simulink model "OFDM_Tx_Rx_InterpDec"  (R2020a)
settings: Solver=FixedStepDiscrete  StartTime=0.0  StopTime=inf  RelTol=1e-3
InitFcn:
  | % Set parameters
  | fs = 200e3;
  | 
  | % Load all required variables
  | load('read_addr_data');
  | load('read_addr_cp');
  | load('read_addr_pream');
  | load('read_addr_rx');
  | load('pilot');
  | load('LTSfreq');
  | load('STSfreq');
  | load('LTSread');
  | load('STSread');
  | load('bpsk');
  | load('qpsk');
  | load('qam16');
values from neighbouring files (symbols this model uses):
  bpsk = [0 0 1 1 1 1 0 0 1 0 1 0 ... (48 elements, 48x1)]    [bpsk.mat]
  qam16 = [12 5 10 3 14 8 1 10 8 7 2 13 ... (48 elements, 48x1)]    [qam16.mat]
  qpsk = [1 2 1 2 2 2 3 1 1 3 1 0 ... (48 elements, 48x1)]    [qpsk.mat]
  STSfreq = [0 0 0 0 0 0 0 0 1 0 0 0 ... (64 elements, 1x64)]    [STSfreq.mat]
undefined symbols (not defined in the file or in its folder): data3, designMultirateFIR, LTSfreq, LTSread, pilot, read_addr_cp, read_addr_data, read_addr_pream, read_addr_rx, STSread
libraries: hdlsllib x58, simulink x42, dspmlti4 x8, dsphdlxfrm x2, dsphdlmathfun x2, dsphdlsigops x1
(part 4 of 5)

== system OFDM_Tx_Rx_InterpDec/OFDMRx/Synchronisation/FineTimingSynch/MatchedFilter/Adder22 ==
  In1 : Inport
  In2 : Inport  Port=2
  Add : Sum  AccumDataTypeStr=fixdt(1,24,14)
  Delay3 : Delay  DelayLength=1
  Out1 : Outport  VectorParamsAs1DForOutWhenUnconnected=off
  wires:
  In2/1 -> Delay3/1
  In1/1 -> Add/1
  Add/1 -> Out1/1
  Delay3/1 -> Add/2

== system OFDM_Tx_Rx_InterpDec/OFDMRx/Synchronisation/FineTimingSynch/MatchedFilter/Adder23 ==
  In1 : Inport
  In2 : Inport  Port=2
  Add : Sum  AccumDataTypeStr=fixdt(1,24,14)
  Delay3 : Delay  DelayLength=1
  Out1 : Outport  VectorParamsAs1DForOutWhenUnconnected=off
  wires:
  In2/1 -> Delay3/1
  In1/1 -> Add/1
  Add/1 -> Out1/1
  Delay3/1 -> Add/2

== system OFDM_Tx_Rx_InterpDec/OFDMRx/Synchronisation/FineTimingSynch/MatchedFilter/Adder24 ==
  In1 : Inport
  In2 : Inport  Port=2
  Add : Sum  AccumDataTypeStr=fixdt(1,24,14)
  Delay3 : Delay  DelayLength=1
  Out1 : Outport  VectorParamsAs1DForOutWhenUnconnected=off
  wires:
  In2/1 -> Delay3/1
  In1/1 -> Add/1
  Add/1 -> Out1/1
  Delay3/1 -> Add/2

== system OFDM_Tx_Rx_InterpDec/OFDMRx/Synchronisation/FineTimingSynch/MatchedFilter/Adder25 ==
  In1 : Inport
  In2 : Inport  Port=2
  Add : Sum  AccumDataTypeStr=fixdt(1,24,14)
  Delay3 : Delay  DelayLength=1
  Out1 : Outport  VectorParamsAs1DForOutWhenUnconnected=off
  wires:
  In2/1 -> Delay3/1
  In1/1 -> Add/1
  Add/1 -> Out1/1
  Delay3/1 -> Add/2

== system OFDM_Tx_Rx_InterpDec/OFDMRx/Synchronisation/FineTimingSynch/MatchedFilter/Adder26 ==
  In1 : Inport
  In2 : Inport  Port=2
  Add : Sum  AccumDataTypeStr=fixdt(1,24,14)
  Delay3 : Delay  DelayLength=1
  Out1 : Outport  VectorParamsAs1DForOutWhenUnconnected=off
  wires:
  In2/1 -> Delay3/1
  In1/1 -> Add/1
  Add/1 -> Out1/1
  Delay3/1 -> Add/2

== system OFDM_Tx_Rx_InterpDec/OFDMRx/Synchronisation/FineTimingSynch/MatchedFilter/Adder27 ==
  In1 : Inport
  In2 : Inport  Port=2
  Add : Sum  AccumDataTypeStr=fixdt(1,24,14)
  Delay3 : Delay  DelayLength=1
  Out1 : Outport  VectorParamsAs1DForOutWhenUnconnected=off
  wires:
  In2/1 -> Delay3/1
  In1/1 -> Add/1
  Add/1 -> Out1/1
  Delay3/1 -> Add/2

== system OFDM_Tx_Rx_InterpDec/OFDMRx/Synchronisation/FineTimingSynch/MatchedFilter/Adder28 ==
  In1 : Inport
  In2 : Inport  Port=2
  Add : Sum
  Delay3 : Delay  DelayLength=1
  Out1 : Outport  VectorParamsAs1DForOutWhenUnconnected=off
  wires:
  In2/1 -> Delay3/1
  In1/1 -> Add/1
  Add/1 -> Out1/1
  Delay3/1 -> Add/2

== system OFDM_Tx_Rx_InterpDec/OFDMRx/Synchronisation/FineTimingSynch/MatchedFilter/Adder29 ==
  In1 : Inport
  In2 : Inport  Port=2
  Add : Sum  AccumDataTypeStr=fixdt(1,24,14)
  Delay3 : Delay  DelayLength=1
  Out1 : Outport  VectorParamsAs1DForOutWhenUnconnected=off
  wires:
  In2/1 -> Delay3/1
  In1/1 -> Add/1
  Add/1 -> Out1/1
  Delay3/1 -> Add/2

== system OFDM_Tx_Rx_InterpDec/OFDMRx/Synchronisation/FineTimingSynch/MatchedFilter/Adder3 ==
  In1 : Inport
  In2 : Inport  Port=2
  Add : Sum  AccumDataTypeStr=fixdt(1,24,14)
  Delay3 : Delay  DelayLength=1
  Out1 : Outport  VectorParamsAs1DForOutWhenUnconnected=off
  wires:
  Delay3/1 -> Add/2
  Add/1 -> Out1/1
  In1/1 -> Add/1
  In2/1 -> Delay3/1

== system OFDM_Tx_Rx_InterpDec/OFDMRx/Synchronisation/FineTimingSynch/MatchedFilter/Adder30 ==
  In1 : Inport
  In2 : Inport  Port=2
  Add : Sum  AccumDataTypeStr=fixdt(1,24,14)
  Delay3 : Delay  DelayLength=1
  Out1 : Outport  VectorParamsAs1DForOutWhenUnconnected=off
  wires:
  In2/1 -> Delay3/1
  In1/1 -> Add/1
  Add/1 -> Out1/1
  Delay3/1 -> Add/2

== system OFDM_Tx_Rx_InterpDec/OFDMRx/Synchronisation/FineTimingSynch/MatchedFilter/Adder31 ==
  In1 : Inport
  In2 : Inport  Port=2
  Add : Sum  AccumDataTypeStr=fixdt(1,24,14)
  Delay3 : Delay  DelayLength=1
  Out1 : Outport  VectorParamsAs1DForOutWhenUnconnected=off
  wires:
  In2/1 -> Delay3/1
  In1/1 -> Add/1
  Add/1 -> Out1/1
  Delay3/1 -> Add/2

== system OFDM_Tx_Rx_InterpDec/OFDMRx/Synchronisation/FineTimingSynch/MatchedFilter/Adder32 ==
  In1 : Inport
  In2 : Inport  Port=2
  Add : Sum  AccumDataTypeStr=fixdt(1,24,14)
  Delay3 : Delay  DelayLength=1
  Out1 : Outport  VectorParamsAs1DForOutWhenUnconnected=off
  wires:
  In2/1 -> Delay3/1
  In1/1 -> Add/1
  Add/1 -> Out1/1
  Delay3/1 -> Add/2

== system OFDM_Tx_Rx_InterpDec/OFDMRx/Synchronisation/FineTimingSynch/MatchedFilter/Adder33 ==
  In1 : Inport
  In2 : Inport  Port=2
  Add : Sum  AccumDataTypeStr=fixdt(1,24,14)
  Delay3 : Delay  DelayLength=1
  Out1 : Outport  VectorParamsAs1DForOutWhenUnconnected=off
  wires:
  In2/1 -> Delay3/1
  In1/1 -> Add/1
  Add/1 -> Out1/1
  Delay3/1 -> Add/2

== system OFDM_Tx_Rx_InterpDec/OFDMRx/Synchronisation/FineTimingSynch/MatchedFilter/Adder34 ==
  In1 : Inport
  In2 : Inport  Port=2
  Add : Sum  AccumDataTypeStr=fixdt(1,24,14)
  Delay3 : Delay  DelayLength=1
  Out1 : Outport  VectorParamsAs1DForOutWhenUnconnected=off
  wires:
  In2/1 -> Delay3/1
  In1/1 -> Add/1
  Add/1 -> Out1/1
  Delay3/1 -> Add/2

== system OFDM_Tx_Rx_InterpDec/OFDMRx/Synchronisation/FineTimingSynch/MatchedFilter/Adder35 ==
  In1 : Inport
  In2 : Inport  Port=2
  Add : Sum  AccumDataTypeStr=fixdt(1,24,14)
  Delay3 : Delay  DelayLength=1
  Out1 : Outport  VectorParamsAs1DForOutWhenUnconnected=off
  wires:
  In2/1 -> Delay3/1
  In1/1 -> Add/1
  Add/1 -> Out1/1
  Delay3/1 -> Add/2

== system OFDM_Tx_Rx_InterpDec/OFDMRx/Synchronisation/FineTimingSynch/MatchedFilter/Adder36 ==
  In1 : Inport
  In2 : Inport  Port=2
  Add : Sum  AccumDataTypeStr=fixdt(1,24,14)
  Delay3 : Delay  DelayLength=1
  Out1 : Outport  VectorParamsAs1DForOutWhenUnconnected=off
  wires:
  In2/1 -> Delay3/1
  In1/1 -> Add/1
  Add/1 -> Out1/1
  Delay3/1 -> Add/2

== system OFDM_Tx_Rx_InterpDec/OFDMRx/Synchronisation/FineTimingSynch/MatchedFilter/Adder37 ==
  In1 : Inport
  In2 : Inport  Port=2
  Add : Sum  AccumDataTypeStr=fixdt(1,24,14)
  Delay3 : Delay  DelayLength=1
  Out1 : Outport  VectorParamsAs1DForOutWhenUnconnected=off
  wires:
  In2/1 -> Delay3/1
  In1/1 -> Add/1
  Add/1 -> Out1/1
  Delay3/1 -> Add/2

== system OFDM_Tx_Rx_InterpDec/OFDMRx/Synchronisation/FineTimingSynch/MatchedFilter/Adder38 ==
  In1 : Inport
  In2 : Inport  Port=2
  Add : Sum  AccumDataTypeStr=fixdt(1,24,14)
  Delay3 : Delay  DelayLength=1
  Out1 : Outport  VectorParamsAs1DForOutWhenUnconnected=off
  wires:
  In2/1 -> Delay3/1
  In1/1 -> Add/1
  Add/1 -> Out1/1
  Delay3/1 -> Add/2

== system OFDM_Tx_Rx_InterpDec/OFDMRx/Synchronisation/FineTimingSynch/MatchedFilter/Adder39 ==
  In1 : Inport
  In2 : Inport  Port=2
  Add : Sum  AccumDataTypeStr=fixdt(1,24,14)
  Delay3 : Delay  DelayLength=1
  Out1 : Outport  VectorParamsAs1DForOutWhenUnconnected=off
  wires:
  In2/1 -> Delay3/1
  In1/1 -> Add/1
  Add/1 -> Out1/1
  Delay3/1 -> Add/2

== system OFDM_Tx_Rx_InterpDec/OFDMRx/Synchronisation/FineTimingSynch/MatchedFilter/Adder4 ==
  In1 : Inport
  In2 : Inport  Port=2
  Add : Sum  AccumDataTypeStr=fixdt(1,24,14)
  Delay3 : Delay  DelayLength=1
  Out1 : Outport  VectorParamsAs1DForOutWhenUnconnected=off
  wires:
  In2/1 -> Delay3/1
  In1/1 -> Add/1
  Add/1 -> Out1/1
  Delay3/1 -> Add/2

== system OFDM_Tx_Rx_InterpDec/OFDMRx/Synchronisation/FineTimingSynch/MatchedFilter/Adder40 ==
  In1 : Inport
  In2 : Inport  Port=2
  Add : Sum  AccumDataTypeStr=fixdt(1,24,14)
  Delay3 : Delay  DelayLength=1
  Out1 : Outport  VectorParamsAs1DForOutWhenUnconnected=off
  wires:
  In2/1 -> Delay3/1
  In1/1 -> Add/1
  Add/1 -> Out1/1
  Delay3/1 -> Add/2

== system OFDM_Tx_Rx_InterpDec/OFDMRx/Synchronisation/FineTimingSynch/MatchedFilter/Adder41 ==
  In1 : Inport
  In2 : Inport  Port=2
  Add : Sum  AccumDataTypeStr=fixdt(1,24,14)
  Delay3 : Delay  DelayLength=1
  Out1 : Outport  VectorParamsAs1DForOutWhenUnconnected=off
  wires:
  In2/1 -> Delay3/1
  In1/1 -> Add/1
  Add/1 -> Out1/1
  Delay3/1 -> Add/2

== system OFDM_Tx_Rx_InterpDec/OFDMRx/Synchronisation/FineTimingSynch/MatchedFilter/Adder42 ==
  In1 : Inport
  In2 : Inport  Port=2
  Add : Sum  AccumDataTypeStr=fixdt(1,24,14)
  Delay3 : Delay  DelayLength=1
  Out1 : Outport  VectorParamsAs1DForOutWhenUnconnected=off
  wires:
  In2/1 -> Delay3/1
  In1/1 -> Add/1
  Add/1 -> Out1/1
  Delay3/1 -> Add/2

== system OFDM_Tx_Rx_InterpDec/OFDMRx/Synchronisation/FineTimingSynch/MatchedFilter/Adder43 ==
  In1 : Inport
  In2 : Inport  Port=2
  Add : Sum  AccumDataTypeStr=fixdt(1,24,14)
  Delay3 : Delay  DelayLength=1
  Out1 : Outport  VectorParamsAs1DForOutWhenUnconnected=off
  wires:
  In2/1 -> Delay3/1
  In1/1 -> Add/1
  Add/1 -> Out1/1
  Delay3/1 -> Add/2

== system OFDM_Tx_Rx_InterpDec/OFDMRx/Synchronisation/FineTimingSynch/MatchedFilter/Adder44 ==
  In1 : Inport
  In2 : Inport  Port=2
  Add : Sum  AccumDataTypeStr=fixdt(1,24,14)
  Delay3 : Delay  DelayLength=1
  Out1 : Outport  VectorParamsAs1DForOutWhenUnconnected=off
  wires:
  In2/1 -> Delay3/1
  In1/1 -> Add/1
  Add/1 -> Out1/1
  Delay3/1 -> Add/2

== system OFDM_Tx_Rx_InterpDec/OFDMRx/Synchronisation/FineTimingSynch/MatchedFilter/Adder45 ==
  In1 : Inport
  In2 : Inport  Port=2
  Add : Sum  AccumDataTypeStr=fixdt(1,24,14)
  Delay3 : Delay  DelayLength=1
  Out1 : Outport  VectorParamsAs1DForOutWhenUnconnected=off
  wires:
  In2/1 -> Delay3/1
  In1/1 -> Add/1
  Add/1 -> Out1/1
  Delay3/1 -> Add/2

== system OFDM_Tx_Rx_InterpDec/OFDMRx/Synchronisation/FineTimingSynch/MatchedFilter/Adder46 ==
  In1 : Inport
  In2 : Inport  Port=2
  Add : Sum  AccumDataTypeStr=fixdt(1,24,14)
  Delay3 : Delay  DelayLength=1
  Out1 : Outport  VectorParamsAs1DForOutWhenUnconnected=off
  wires:
  In2/1 -> Delay3/1
  In1/1 -> Add/1
  Add/1 -> Out1/1
  Delay3/1 -> Add/2

== system OFDM_Tx_Rx_InterpDec/OFDMRx/Synchronisation/FineTimingSynch/MatchedFilter/Adder47 ==
  In1 : Inport
  In2 : Inport  Port=2
  Add : Sum  AccumDataTypeStr=fixdt(1,24,14)
  Delay3 : Delay  DelayLength=1
  Out1 : Outport  VectorParamsAs1DForOutWhenUnconnected=off
  wires:
  In2/1 -> Delay3/1
  In1/1 -> Add/1
  Add/1 -> Out1/1
  Delay3/1 -> Add/2

== system OFDM_Tx_Rx_InterpDec/OFDMRx/Synchronisation/FineTimingSynch/MatchedFilter/Adder48 ==
  In1 : Inport
  In2 : Inport  Port=2
  Add : Sum  AccumDataTypeStr=fixdt(1,24,14)
  Delay3 : Delay  DelayLength=1
  Out1 : Outport  VectorParamsAs1DForOutWhenUnconnected=off
  wires:
  In2/1 -> Delay3/1
  In1/1 -> Add/1
  Add/1 -> Out1/1
  Delay3/1 -> Add/2

== system OFDM_Tx_Rx_InterpDec/OFDMRx/Synchronisation/FineTimingSynch/MatchedFilter/Adder49 ==
  In1 : Inport
  In2 : Inport  Port=2
  Add : Sum  AccumDataTypeStr=fixdt(1,24,14)
  Delay3 : Delay  DelayLength=1
  Out1 : Outport  VectorParamsAs1DForOutWhenUnconnected=off
  wires:
  In2/1 -> Delay3/1
  In1/1 -> Add/1
  Add/1 -> Out1/1
  Delay3/1 -> Add/2

== system OFDM_Tx_Rx_InterpDec/OFDMRx/Synchronisation/FineTimingSynch/MatchedFilter/Adder5 ==
  In1 : Inport
  In2 : Inport  Port=2
  Add : Sum  AccumDataTypeStr=fixdt(1,24,14)
  Delay3 : Delay  DelayLength=1
  Out1 : Outport  VectorParamsAs1DForOutWhenUnconnected=off
  wires:
  Delay3/1 -> Add/2
  Add/1 -> Out1/1
  In1/1 -> Add/1
  In2/1 -> Delay3/1

== system OFDM_Tx_Rx_InterpDec/OFDMRx/Synchronisation/FineTimingSynch/MatchedFilter/Adder50 ==
  In1 : Inport
  In2 : Inport  Port=2
  Add : Sum  AccumDataTypeStr=fixdt(1,24,14)
  Delay3 : Delay  DelayLength=1
  Out1 : Outport  VectorParamsAs1DForOutWhenUnconnected=off
  wires:
  In2/1 -> Delay3/1
  In1/1 -> Add/1
  Add/1 -> Out1/1
  Delay3/1 -> Add/2

== system OFDM_Tx_Rx_InterpDec/OFDMRx/Synchronisation/FineTimingSynch/MatchedFilter/Adder51 ==
  In1 : Inport
  In2 : Inport  Port=2
  Add : Sum  AccumDataTypeStr=fixdt(1,24,14)
  Delay3 : Delay  DelayLength=1
  Out1 : Outport  VectorParamsAs1DForOutWhenUnconnected=off
  wires:
  In2/1 -> Delay3/1
  In1/1 -> Add/1
  Add/1 -> Out1/1
  Delay3/1 -> Add/2

== system OFDM_Tx_Rx_InterpDec/OFDMRx/Synchronisation/FineTimingSynch/MatchedFilter/Adder52 ==
  In1 : Inport
  In2 : Inport  Port=2
  Add : Sum  AccumDataTypeStr=fixdt(1,24,14)
  Delay3 : Delay  DelayLength=1
  Out1 : Outport  VectorParamsAs1DForOutWhenUnconnected=off
  wires:
  In2/1 -> Delay3/1
  In1/1 -> Add/1
  Add/1 -> Out1/1
  Delay3/1 -> Add/2

== system OFDM_Tx_Rx_InterpDec/OFDMRx/Synchronisation/FineTimingSynch/MatchedFilter/Adder53 ==
  In1 : Inport
  In2 : Inport  Port=2
  Add : Sum  AccumDataTypeStr=fixdt(1,24,14)
  Delay3 : Delay  DelayLength=1
  Out1 : Outport  VectorParamsAs1DForOutWhenUnconnected=off
  wires:
  In2/1 -> Delay3/1
  In1/1 -> Add/1
  Add/1 -> Out1/1
  Delay3/1 -> Add/2

== system OFDM_Tx_Rx_InterpDec/OFDMRx/Synchronisation/FineTimingSynch/MatchedFilter/Adder54 ==
  In1 : Inport
  In2 : Inport  Port=2
  Add : Sum  AccumDataTypeStr=fixdt(1,24,14)
  Delay3 : Delay  DelayLength=1
  Out1 : Outport  VectorParamsAs1DForOutWhenUnconnected=off
  wires:
  In2/1 -> Delay3/1
  In1/1 -> Add/1
  Add/1 -> Out1/1
  Delay3/1 -> Add/2

== system OFDM_Tx_Rx_InterpDec/OFDMRx/Synchronisation/FineTimingSynch/MatchedFilter/Adder55 ==
  In1 : Inport
  In2 : Inport  Port=2
  Add : Sum  AccumDataTypeStr=fixdt(1,24,14)
  Delay3 : Delay  DelayLength=1
  Out1 : Outport  VectorParamsAs1DForOutWhenUnconnected=off
  wires:
  In2/1 -> Delay3/1
  In1/1 -> Add/1
  Add/1 -> Out1/1
  Delay3/1 -> Add/2

== system OFDM_Tx_Rx_InterpDec/OFDMRx/Synchronisation/FineTimingSynch/MatchedFilter/Adder56 ==
  In1 : Inport
  In2 : Inport  Port=2
  Add : Sum  AccumDataTypeStr=fixdt(1,24,14)
  Delay3 : Delay  DelayLength=1
  Out1 : Outport  VectorParamsAs1DForOutWhenUnconnected=off
  wires:
  In2/1 -> Delay3/1
  In1/1 -> Add/1
  Add/1 -> Out1/1
  Delay3/1 -> Add/2

== system OFDM_Tx_Rx_InterpDec/OFDMRx/Synchronisation/FineTimingSynch/MatchedFilter/Adder57 ==
  In1 : Inport
  In2 : Inport  Port=2
  Add : Sum  AccumDataTypeStr=fixdt(1,24,14)
  Delay3 : Delay  DelayLength=1
  Out1 : Outport  VectorParamsAs1DForOutWhenUnconnected=off
  wires:
  In2/1 -> Delay3/1
  In1/1 -> Add/1
  Add/1 -> Out1/1
  Delay3/1 -> Add/2

== system OFDM_Tx_Rx_InterpDec/OFDMRx/Synchronisation/FineTimingSynch/MatchedFilter/Adder58 ==
  In1 : Inport
  In2 : Inport  Port=2
  Add : Sum  AccumDataTypeStr=fixdt(1,24,14)
  Delay3 : Delay  DelayLength=1
  Out1 : Outport  VectorParamsAs1DForOutWhenUnconnected=off
  wires:
  In2/1 -> Delay3/1
  In1/1 -> Add/1
  Add/1 -> Out1/1
  Delay3/1 -> Add/2

== system OFDM_Tx_Rx_InterpDec/OFDMRx/Synchronisation/FineTimingSynch/MatchedFilter/Adder59 ==
  In1 : Inport
  In2 : Inport  Port=2
  Add : Sum  AccumDataTypeStr=fixdt(1,24,14)
  Delay3 : Delay  DelayLength=1
  Out1 : Outport  VectorParamsAs1DForOutWhenUnconnected=off
  wires:
  In2/1 -> Delay3/1
  In1/1 -> Add/1
  Add/1 -> Out1/1
  Delay3/1 -> Add/2

== system OFDM_Tx_Rx_InterpDec/OFDMRx/Synchronisation/FineTimingSynch/MatchedFilter/Adder6 ==
  In1 : Inport
  In2 : Inport  Port=2
  Add : Sum  AccumDataTypeStr=fixdt(1,24,14)
  Delay3 : Delay  DelayLength=1
  Out1 : Outport  VectorParamsAs1DForOutWhenUnconnected=off
  wires:
  In2/1 -> Delay3/1
  In1/1 -> Add/1
  Add/1 -> Out1/1
  Delay3/1 -> Add/2

== system OFDM_Tx_Rx_InterpDec/OFDMRx/Synchronisation/FineTimingSynch/MatchedFilter/Adder60 ==
  In1 : Inport
  In2 : Inport  Port=2
  Add : Sum  AccumDataTypeStr=fixdt(1,24,14)
  Delay3 : Delay  DelayLength=1
  Out1 : Outport  VectorParamsAs1DForOutWhenUnconnected=off
  wires:
  In2/1 -> Delay3/1
  In1/1 -> Add/1
  Add/1 -> Out1/1
  Delay3/1 -> Add/2

== system OFDM_Tx_Rx_InterpDec/OFDMRx/Synchronisation/FineTimingSynch/MatchedFilter/Adder61 ==
  In1 : Inport
  In2 : Inport  Port=2
  Add : Sum  AccumDataTypeStr=fixdt(1,24,14)
  Delay3 : Delay  DelayLength=1
  Out1 : Outport  VectorParamsAs1DForOutWhenUnconnected=off
  wires:
  In2/1 -> Delay3/1
  In1/1 -> Add/1
  Add/1 -> Out1/1
  Delay3/1 -> Add/2

== system OFDM_Tx_Rx_InterpDec/OFDMRx/Synchronisation/FineTimingSynch/MatchedFilter/Adder62 ==
  In1 : Inport
  In2 : Inport  Port=2
  Add : Sum  AccumDataTypeStr=fixdt(1,24,14)
  Delay3 : Delay  DelayLength=1
  Out1 : Outport  VectorParamsAs1DForOutWhenUnconnected=off
  wires:
  In2/1 -> Delay3/1
  In1/1 -> Add/1
  Add/1 -> Out1/1
  Delay3/1 -> Add/2

== system OFDM_Tx_Rx_InterpDec/OFDMRx/Synchronisation/FineTimingSynch/MatchedFilter/Adder7 ==
  In1 : Inport
  In2 : Inport  Port=2
  Add : Sum  AccumDataTypeStr=fixdt(1,24,14)
  Delay3 : Delay  DelayLength=1
  Out1 : Outport  VectorParamsAs1DForOutWhenUnconnected=off
  wires:
  Delay3/1 -> Add/2
  Add/1 -> Out1/1
  In1/1 -> Add/1
  In2/1 -> Delay3/1

== system OFDM_Tx_Rx_InterpDec/OFDMRx/Synchronisation/FineTimingSynch/MatchedFilter/Adder8 ==
  In1 : Inport
  In2 : Inport  Port=2
  Add : Sum  AccumDataTypeStr=fixdt(1,24,14)
  Delay3 : Delay  DelayLength=1
  Out1 : Outport  VectorParamsAs1DForOutWhenUnconnected=off
  wires:
  In2/1 -> Delay3/1
  In1/1 -> Add/1
  Add/1 -> Out1/1
  Delay3/1 -> Add/2

== system OFDM_Tx_Rx_InterpDec/OFDMRx/Synchronisation/FineTimingSynch/MatchedFilter/Adder9 ==
  In1 : Inport
  In2 : Inport  Port=2
  Add : Sum  AccumDataTypeStr=fixdt(1,24,14)
  Delay3 : Delay  DelayLength=1
  Out1 : Outport  VectorParamsAs1DForOutWhenUnconnected=off
  wires:
  Delay3/1 -> Add/2
  Add/1 -> Out1/1
  In1/1 -> Add/1
  In2/1 -> Delay3/1

== system OFDM_Tx_Rx_InterpDec/OFDMRx/Synchronisation/FineTimingSynch/MatchedFilter/Subsystem ==
  MatchedIn : Inport
  Add : Sum  OutDataTypeStr=fixdt(1,18,14)
  Add1 : Sum  Inputs=+-  OutDataTypeStr=fixdt(1,18,14)
  Complex to Real-Imag : ComplexToRealImag
  Real-Imag to Complex : RealImagToComplex
  Unary Minus : UnaryMinus
  Out1 : Outport
  wires:
  Real-Imag to Complex/1 -> Out1/1
  MatchedIn/1 -> Complex to Real-Imag/1
  Add1/1 -> Real-Imag to Complex/1
  Complex to Real-Imag/2 -> Add/2, Add1/1
  Complex to Real-Imag/1 -> Add/1, Add1/2
  Add/1 -> Unary Minus/1
  Unary Minus/1 -> Real-Imag to Complex/2

== system OFDM_Tx_Rx_InterpDec/OFDMRx/Synchronisation/FineTimingSynch/MatchedFilter/Subsystem1 ==
  MatchedIn : Inport
  Add : Sum  OutDataTypeStr=fixdt(1,18,14)
  Add1 : Sum  Inputs=+-  OutDataTypeStr=fixdt(1,18,14)
  Complex to Real-Imag : ComplexToRealImag
  Real-Imag to Complex : RealImagToComplex
  Out1 : Outport
  wires:
  Complex to Real-Imag/2 -> Add1/1, Add/2
  Add/1 -> Real-Imag to Complex/1
  Add1/1 -> Real-Imag to Complex/2
  Complex to Real-Imag/1 -> Add1/2, Add/1
  MatchedIn/1 -> Complex to Real-Imag/1
  Real-Imag to Complex/1 -> Out1/1

== system OFDM_Tx_Rx_InterpDec/OFDMRx/Synchronisation/FineTimingSynch/MatchedFilter/Subsystem10 ==
  MatchedIn : Inport
  Add : Sum  OutDataTypeStr=fixdt(1,18,14)
  Add1 : Sum  Inputs=+-  OutDataTypeStr=fixdt(1,18,14)
  Complex to Real-Imag : ComplexToRealImag
  Real-Imag to Complex : RealImagToComplex
  Unary Minus : UnaryMinus
  Out1 : Outport
  wires:
  Unary Minus/1 -> Real-Imag to Complex/2
  Add/1 -> Unary Minus/1
  Complex to Real-Imag/1 -> Add1/2, Add/1
  Complex to Real-Imag/2 -> Add1/1, Add/2
  Add1/1 -> Real-Imag to Complex/1
  MatchedIn/1 -> Complex to Real-Imag/1
  Real-Imag to Complex/1 -> Out1/1

== system OFDM_Tx_Rx_InterpDec/OFDMRx/Synchronisation/FineTimingSynch/MatchedFilter/Subsystem11 ==
  MatchedIn : Inport
  Add : Sum  OutDataTypeStr=fixdt(1,18,14)
  Add1 : Sum  Inputs=+-  OutDataTypeStr=fixdt(1,18,14)
  Complex to Real-Imag : ComplexToRealImag
  Real-Imag to Complex : RealImagToComplex
  Out1 : Outport
  wires:
  Real-Imag to Complex/1 -> Out1/1
  MatchedIn/1 -> Complex to Real-Imag/1
  Complex to Real-Imag/1 -> Add/1, Add1/2
  Add1/1 -> Real-Imag to Complex/2
  Add/1 -> Real-Imag to Complex/1
  Complex to Real-Imag/2 -> Add/2, Add1/1

== system OFDM_Tx_Rx_InterpDec/OFDMRx/Synchronisation/FineTimingSynch/MatchedFilter/Subsystem12 ==
  MatchedIn : Inport
  Add : Sum  OutDataTypeStr=fixdt(1,18,14)
  Add1 : Sum  Inputs=+-  OutDataTypeStr=fixdt(1,18,14)
  Complex to Real-Imag : ComplexToRealImag
  Real-Imag to Complex : RealImagToComplex
  Out1 : Outport
  wires:
  Real-Imag to Complex/1 -> Out1/1
  MatchedIn/1 -> Complex to Real-Imag/1
  Complex to Real-Imag/1 -> Add/1, Add1/2
  Add1/1 -> Real-Imag to Complex/2
  Add/1 -> Real-Imag to Complex/1
  Complex to Real-Imag/2 -> Add/2, Add1/1

== system OFDM_Tx_Rx_InterpDec/OFDMRx/Synchronisation/FineTimingSynch/MatchedFilter/Subsystem13 ==
  MatchedIn : Inport
  Add : Sum  OutDataTypeStr=fixdt(1,18,14)
  Add1 : Sum  Inputs=+-  OutDataTypeStr=fixdt(1,18,14)
  Complex to Real-Imag : ComplexToRealImag
  Real-Imag to Complex : RealImagToComplex
  Unary Minus : UnaryMinus
  Out1 : Outport
  wires:
  Complex to Real-Imag/2 -> Add1/2, Add/2
  Add/1 -> Unary Minus/1
  Add1/1 -> Real-Imag to Complex/2
  Complex to Real-Imag/1 -> Add1/1, Add/1
  MatchedIn/1 -> Complex to Real-Imag/1
  Real-Imag to Complex/1 -> Out1/1
  Unary Minus/1 -> Real-Imag to Complex/1

== system OFDM_Tx_Rx_InterpDec/OFDMRx/Synchronisation/FineTimingSynch/MatchedFilter/Subsystem14 ==
  MatchedIn : Inport
  Add : Sum  OutDataTypeStr=fixdt(1,18,14)
  Add1 : Sum  Inputs=+-  OutDataTypeStr=fixdt(1,18,14)
  Complex to Real-Imag : ComplexToRealImag
  Real-Imag to Complex : RealImagToComplex
  Out1 : Outport
  wires:
  Real-Imag to Complex/1 -> Out1/1
  MatchedIn/1 -> Complex to Real-Imag/1
  Complex to Real-Imag/1 -> Add/1, Add1/2
  Add1/1 -> Real-Imag to Complex/2
  Add/1 -> Real-Imag to Complex/1
  Complex to Real-Imag/2 -> Add/2, Add1/1

== system OFDM_Tx_Rx_InterpDec/OFDMRx/Synchronisation/FineTimingSynch/MatchedFilter/Subsystem15 ==
  MatchedIn : Inport
  Add : Sum  OutDataTypeStr=fixdt(1,18,14)
  Add1 : Sum  Inputs=+-  OutDataTypeStr=fixdt(1,18,14)
  Complex to Real-Imag : ComplexToRealImag
  Real-Imag to Complex : RealImagToComplex
  Out1 : Outport
  wires:
  Real-Imag to Complex/1 -> Out1/1
  MatchedIn/1 -> Complex to Real-Imag/1
  Complex to Real-Imag/1 -> Add/1, Add1/2
  Add1/1 -> Real-Imag to Complex/2
  Add/1 -> Real-Imag to Complex/1
  Complex to Real-Imag/2 -> Add/2, Add1/1

== system OFDM_Tx_Rx_InterpDec/OFDMRx/Synchronisation/FineTimingSynch/MatchedFilter/Subsystem16 ==
  MatchedIn : Inport
  Add : Sum  OutDataTypeStr=fixdt(1,18,14)
  Add1 : Sum  Inputs=+-  OutDataTypeStr=fixdt(1,18,14)
  Complex to Real-Imag : ComplexToRealImag
  Real-Imag to Complex : RealImagToComplex
  Out1 : Outport
  wires:
  Add/1 -> Real-Imag to Complex/2
  Add1/1 -> Real-Imag to Complex/1
  Complex to Real-Imag/2 -> Add/2, Add1/2
  Complex to Real-Imag/1 -> Add/1, Add1/1
  MatchedIn/1 -> Complex to Real-Imag/1
  Real-Imag to Complex/1 -> Out1/1

== system OFDM_Tx_Rx_InterpDec/OFDMRx/Synchronisation/FineTimingSynch/MatchedFilter/Subsystem17 ==
  MatchedIn : Inport
  Add : Sum  OutDataTypeStr=fixdt(1,18,14)
  Add1 : Sum  Inputs=+-  OutDataTypeStr=fixdt(1,18,14)
  Complex to Real-Imag : ComplexToRealImag
  Real-Imag to Complex : RealImagToComplex
  Unary Minus : UnaryMinus
  Out1 : Outport
  wires:
  Unary Minus/1 -> Real-Imag to Complex/1
  Real-Imag to Complex/1 -> Out1/1
  MatchedIn/1 -> Complex to Real-Imag/1
  Complex to Real-Imag/1 -> Add/1, Add1/1
  Add1/1 -> Real-Imag to Complex/2
  Add/1 -> Unary Minus/1
  Complex to Real-Imag/2 -> Add/2, Add1/2

== system OFDM_Tx_Rx_InterpDec/OFDMRx/Synchronisation/FineTimingSynch/MatchedFilter/Subsystem18 ==
  MatchedIn : Inport
  Add : Sum  OutDataTypeStr=fixdt(1,18,14)
  Add1 : Sum  Inputs=+-  OutDataTypeStr=fixdt(1,18,14)
  Complex to Real-Imag : ComplexToRealImag
  Real-Imag to Complex : RealImagToComplex
  Unary Minus : UnaryMinus
  Out1 : Outport
  wires:
  Unary Minus/1 -> Real-Imag to Complex/1
  Real-Imag to Complex/1 -> Out1/1
  MatchedIn/1 -> Complex to Real-Imag/1
  Complex to Real-Imag/1 -> Add/1, Add1/1
  Add1/1 -> Real-Imag to Complex/2
  Add/1 -> Unary Minus/1
  Complex to Real-Imag/2 -> Add/2, Add1/2

== system OFDM_Tx_Rx_InterpDec/OFDMRx/Synchronisation/FineTimingSynch/MatchedFilter/Subsystem19 ==
  MatchedIn : Inport
  Add : Sum  OutDataTypeStr=fixdt(1,18,14)
  Add1 : Sum  Inputs=+-  OutDataTypeStr=fixdt(1,18,14)
  Complex to Real-Imag : ComplexToRealImag
  Real-Imag to Complex : RealImagToComplex
  Out1 : Outport
  wires:
  Add/1 -> Real-Imag to Complex/2
  Add1/1 -> Real-Imag to Complex/1
  Complex to Real-Imag/2 -> Add/2, Add1/2
  Complex to Real-Imag/1 -> Add/1, Add1/1
  MatchedIn/1 -> Complex to Real-Imag/1
  Real-Imag to Complex/1 -> Out1/1

== system OFDM_Tx_Rx_InterpDec/OFDMRx/Synchronisation/FineTimingSynch/MatchedFilter/Subsystem2 ==
  MatchedIn : Inport
  Add : Sum  OutDataTypeStr=fixdt(1,18,14)
  Add1 : Sum  Inputs=+-  OutDataTypeStr=fixdt(1,18,14)
  Complex to Real-Imag : ComplexToRealImag
  Real-Imag to Complex : RealImagToComplex
  Out1 : Outport
  wires:
  Real-Imag to Complex/1 -> Out1/1
  MatchedIn/1 -> Complex to Real-Imag/1
  Complex to Real-Imag/1 -> Add1/1, Add/1
  Complex to Real-Imag/2 -> Add1/2, Add/2
  Add1/1 -> Real-Imag to Complex/1
  Add/1 -> Real-Imag to Complex/2

== system OFDM_Tx_Rx_InterpDec/OFDMRx/Synchronisation/FineTimingSynch/MatchedFilter/Subsystem20 ==
  MatchedIn : Inport
  Add : Sum  OutDataTypeStr=fixdt(1,18,14)
  Add1 : Sum  Inputs=+-  OutDataTypeStr=fixdt(1,18,14)
  Complex to Real-Imag : ComplexToRealImag
  Real-Imag to Complex : RealImagToComplex
  Out1 : Outport
  wires:
  Add/1 -> Real-Imag to Complex/2
  Add1/1 -> Real-Imag to Complex/1
  Complex to Real-Imag/2 -> Add/2, Add1/2
  Complex to Real-Imag/1 -> Add/1, Add1/1
  MatchedIn/1 -> Complex to Real-Imag/1
  Real-Imag to Complex/1 -> Out1/1

== system OFDM_Tx_Rx_InterpDec/OFDMRx/Synchronisation/FineTimingSynch/MatchedFilter/Subsystem21 ==
  MatchedIn : Inport
  Add : Sum  OutDataTypeStr=fixdt(1,18,14)
  Add1 : Sum  Inputs=+-  OutDataTypeStr=fixdt(1,18,14)
  Complex to Real-Imag : ComplexToRealImag
  Real-Imag to Complex : RealImagToComplex
  Unary Minus : UnaryMinus
  Out1 : Outport
  wires:
  Unary Minus/1 -> Real-Imag to Complex/1
  Real-Imag to Complex/1 -> Out1/1
  MatchedIn/1 -> Complex to Real-Imag/1
  Complex to Real-Imag/1 -> Add/1, Add1/1
  Add1/1 -> Real-Imag to Complex/2
  Add/1 -> Unary Minus/1
  Complex to Real-Imag/2 -> Add/2, Add1/2

== system OFDM_Tx_Rx_InterpDec/OFDMRx/Synchronisation/FineTimingSynch/MatchedFilter/Subsystem22 ==
  MatchedIn : Inport
  Add : Sum  OutDataTypeStr=fixdt(1,18,14)
  Add1 : Sum  Inputs=+-  OutDataTypeStr=fixdt(1,18,14)
  Complex to Real-Imag : ComplexToRealImag
  Real-Imag to Complex : RealImagToComplex
  Unary Minus : UnaryMinus
  Out1 : Outport
  wires:
  Unary Minus/1 -> Real-Imag to Complex/2
  Add/1 -> Unary Minus/1
  Complex to Real-Imag/1 -> Add1/2, Add/1
  Complex to Real-Imag/2 -> Add1/1, Add/2
  Add1/1 -> Real-Imag to Complex/1
  MatchedIn/1 -> Complex to Real-Imag/1
  Real-Imag to Complex/1 -> Out1/1

== system OFDM_Tx_Rx_InterpDec/OFDMRx/Synchronisation/FineTimingSynch/MatchedFilter/Subsystem23 ==
  MatchedIn : Inport
  Add : Sum  OutDataTypeStr=fixdt(1,18,14)
  Add1 : Sum  Inputs=+-  OutDataTypeStr=fixdt(1,18,14)
  Complex to Real-Imag : ComplexToRealImag
  Real-Imag to Complex : RealImagToComplex
  Unary Minus : UnaryMinus
  Out1 : Outport
  wires:
  Real-Imag to Complex/1 -> Out1/1
  MatchedIn/1 -> Complex to Real-Imag/1
  Add1/1 -> Real-Imag to Complex/1
  Complex to Real-Imag/2 -> Add/2, Add1/1
  Complex to Real-Imag/1 -> Add/1, Add1/2
  Add/1 -> Unary Minus/1
  Unary Minus/1 -> Real-Imag to Complex/2

== system OFDM_Tx_Rx_InterpDec/OFDMRx/Synchronisation/FineTimingSynch/MatchedFilter/Subsystem24 ==
  MatchedIn : Inport
  Add : Sum  OutDataTypeStr=fixdt(1,18,14)
  Add1 : Sum  Inputs=+-  OutDataTypeStr=fixdt(1,18,14)
  Complex to Real-Imag : ComplexToRealImag
  Real-Imag to Complex : RealImagToComplex
  Unary Minus : UnaryMinus
  Out1 : Outport
  wires:
  Unary Minus/1 -> Real-Imag to Complex/2
  Add/1 -> Unary Minus/1
  Complex to Real-Imag/1 -> Add1/2, Add/1
  Complex to Real-Imag/2 -> Add1/1, Add/2
  Add1/1 -> Real-Imag to Complex/1
  MatchedIn/1 -> Complex to Real-Imag/1
  Real-Imag to Complex/1 -> Out1/1

== system OFDM_Tx_Rx_InterpDec/OFDMRx/Synchronisation/FineTimingSynch/MatchedFilter/Subsystem25 ==
  MatchedIn : Inport
  Add : Sum  OutDataTypeStr=fixdt(1,18,14)
  Add1 : Sum  Inputs=+-  OutDataTypeStr=fixdt(1,18,14)
  Complex to Real-Imag : ComplexToRealImag
  Real-Imag to Complex : RealImagToComplex
  Unary Minus : UnaryMinus
  Out1 : Outport
  wires:
  Real-Imag to Complex/1 -> Out1/1
  MatchedIn/1 -> Complex to Real-Imag/1
  Add1/1 -> Real-Imag to Complex/1
  Complex to Real-Imag/2 -> Add/2, Add1/1
  Complex to Real-Imag/1 -> Add/1, Add1/2
  Add/1 -> Unary Minus/1
  Unary Minus/1 -> Real-Imag to Complex/2

== system OFDM_Tx_Rx_InterpDec/OFDMRx/Synchronisation/FineTimingSynch/MatchedFilter/Subsystem26 ==
  MatchedIn : Inport
  Add : Sum  OutDataTypeStr=fixdt(1,18,14)
  Add1 : Sum  Inputs=+-  OutDataTypeStr=fixdt(1,18,14)
  Complex to Real-Imag : ComplexToRealImag
  Real-Imag to Complex : RealImagToComplex
  Out1 : Outport
  wires:
  Real-Imag to Complex/1 -> Out1/1
  MatchedIn/1 -> Complex to Real-Imag/1
  Complex to Real-Imag/1 -> Add/1, Add1/2
  Add1/1 -> Real-Imag to Complex/2
  Add/1 -> Real-Imag to Complex/1
  Complex to Real-Imag/2 -> Add/2, Add1/1

== system OFDM_Tx_Rx_InterpDec/OFDMRx/Synchronisation/FineTimingSynch/MatchedFilter/Subsystem27 ==
  MatchedIn : Inport
  Add : Sum  OutDataTypeStr=fixdt(1,18,14)
  Add1 : Sum  Inputs=+-  OutDataTypeStr=fixdt(1,18,14)
  Complex to Real-Imag : ComplexToRealImag
  Real-Imag to Complex : RealImagToComplex
  Unary Minus : UnaryMinus
  Out1 : Outport
  wires:
  Unary Minus/1 -> Real-Imag to Complex/1
  Real-Imag to Complex/1 -> Out1/1
  MatchedIn/1 -> Complex to Real-Imag/1
  Complex to Real-Imag/1 -> Add/1, Add1/1
  Add1/1 -> Real-Imag to Complex/2
  Add/1 -> Unary Minus/1
  Complex to Real-Imag/2 -> Add/2, Add1/2

== system OFDM_Tx_Rx_InterpDec/OFDMRx/Synchronisation/FineTimingSynch/MatchedFilter/Subsystem28 ==
  MatchedIn : Inport
  Add : Sum  OutDataTypeStr=fixdt(1,18,14)
  Add1 : Sum  Inputs=+-  OutDataTypeStr=fixdt(1,18,14)
  Complex to Real-Imag : ComplexToRealImag
  Real-Imag to Complex : RealImagToComplex
  Unary Minus : UnaryMinus
  Out1 : Outport
  wires:
  Unary Minus/1 -> Real-Imag to Complex/1
  Real-Imag to Complex/1 -> Out1/1
  MatchedIn/1 -> Complex to Real-Imag/1
  Complex to Real-Imag/1 -> Add/1, Add1/1
  Add1/1 -> Real-Imag to Complex/2
  Add/1 -> Unary Minus/1
  Complex to Real-Imag/2 -> Add/2, Add1/2

== system OFDM_Tx_Rx_InterpDec/OFDMRx/Synchronisation/FineTimingSynch/MatchedFilter/Subsystem29 ==
  MatchedIn : Inport
  Add : Sum  OutDataTypeStr=fixdt(1,18,14)
  Add1 : Sum  Inputs=+-  OutDataTypeStr=fixdt(1,18,14)
  Complex to Real-Imag : ComplexToRealImag
  Real-Imag to Complex : RealImagToComplex
  Out1 : Outport
  wires:
  Add/1 -> Real-Imag to Complex/2
  Add1/1 -> Real-Imag to Complex/1
  Complex to Real-Imag/2 -> Add/2, Add1/2
  Complex to Real-Imag/1 -> Add/1, Add1/1
  MatchedIn/1 -> Complex to Real-Imag/1
  Real-Imag to Complex/1 -> Out1/1

== system OFDM_Tx_Rx_InterpDec/OFDMRx/Synchronisation/FineTimingSynch/MatchedFilter/Subsystem3 ==
  MatchedIn : Inport
  Add : Sum  OutDataTypeStr=fixdt(1,18,14)
  Add1 : Sum  Inputs=+-  OutDataTypeStr=fixdt(1,18,14)
  Complex to Real-Imag : ComplexToRealImag
  Real-Imag to Complex : RealImagToComplex
  Out1 : Outport
  wires:
  Add/1 -> Real-Imag to Complex/2
  Add1/1 -> Real-Imag to Complex/1
  Complex to Real-Imag/2 -> Add/2, Add1/2
  Complex to Real-Imag/1 -> Add/1, Add1/1
  MatchedIn/1 -> Complex to Real-Imag/1
  Real-Imag to Complex/1 -> Out1/1

== system OFDM_Tx_Rx_InterpDec/OFDMRx/Synchronisation/FineTimingSynch/MatchedFilter/Subsystem30 ==
  MatchedIn : Inport
  Add : Sum  OutDataTypeStr=fixdt(1,18,14)
  Add1 : Sum  Inputs=+-  OutDataTypeStr=fixdt(1,18,14)
  Complex to Real-Imag : ComplexToRealImag
  Real-Imag to Complex : RealImagToComplex
  Out1 : Outport
  wires:
  Add/1 -> Real-Imag to Complex/2
  Add1/1 -> Real-Imag to Complex/1
  Complex to Real-Imag/2 -> Add/2, Add1/2
  Complex to Real-Imag/1 -> Add/1, Add1/1
  MatchedIn/1 -> Complex to Real-Imag/1
  Real-Imag to Complex/1 -> Out1/1

== system OFDM_Tx_Rx_InterpDec/OFDMRx/Synchronisation/FineTimingSynch/MatchedFilter/Subsystem31 ==
  In1 : Inport
  Complex to Real-Imag : ComplexToRealImag
  Real-Imag to Complex : RealImagToComplex
  Unary Minus : UnaryMinus
  Unary Minus1 : UnaryMinus
  Out1 : Outport
  wires:
  Unary Minus/1 -> Real-Imag to Complex/1
  Real-Imag to Complex/1 -> Out1/1
  Unary Minus1/1 -> Real-Imag to Complex/2
  Complex to Real-Imag/2 -> Unary Minus1/1
  Complex to Real-Imag/1 -> Unary Minus/1
  In1/1 -> Complex to Real-Imag/1

== system OFDM_Tx_Rx_InterpDec/OFDMRx/Synchronisation/FineTimingSynch/MatchedFilter/Subsystem32 ==
  MatchedIn : Inport
  Add : Sum  OutDataTypeStr=fixdt(1,18,14)
  Add1 : Sum  Inputs=+-  OutDataTypeStr=fixdt(1,18,14)
  Complex to Real-Imag : ComplexToRealImag
  Real-Imag to Complex : RealImagToComplex
  Out1 : Outport
  wires:
  Real-Imag to Complex/1 -> Out1/1
  MatchedIn/1 -> Complex to Real-Imag/1
  Complex to Real-Imag/1 -> Add/1, Add1/2
  Add1/1 -> Real-Imag to Complex/2
  Add/1 -> Real-Imag to Complex/1
  Complex to Real-Imag/2 -> Add/2, Add1/1

== system OFDM_Tx_Rx_InterpDec/OFDMRx/Synchronisation/FineTimingSynch/MatchedFilter/Subsystem33 ==
  MatchedIn : Inport
  Add : Sum  OutDataTypeStr=fixdt(1,18,14)
  Add1 : Sum  Inputs=+-  OutDataTypeStr=fixdt(1,18,14)
  Complex to Real-Imag : ComplexToRealImag
  Real-Imag to Complex : RealImagToComplex
  Out1 : Outport
  wires:
  Real-Imag to Complex/1 -> Out1/1
  MatchedIn/1 -> Complex to Real-Imag/1
  Complex to Real-Imag/1 -> Add/1, Add1/2
  Add1/1 -> Real-Imag to Complex/2
  Add/1 -> Real-Imag to Complex/1
  Complex to Real-Imag/2 -> Add/2, Add1/1

== system OFDM_Tx_Rx_InterpDec/OFDMRx/Synchronisation/FineTimingSynch/MatchedFilter/Subsystem34 ==
  MatchedIn : Inport
  Add : Sum  OutDataTypeStr=fixdt(1,18,14)
  Add1 : Sum  Inputs=+-  OutDataTypeStr=fixdt(1,18,14)
  Complex to Real-Imag : ComplexToRealImag
  Real-Imag to Complex : RealImagToComplex
  Unary Minus : UnaryMinus
  Out1 : Outport
  wires:
  Unary Minus/1 -> Real-Imag to Complex/2
  Add/1 -> Unary Minus/1
  Complex to Real-Imag/1 -> Add1/2, Add/1
  Complex to Real-Imag/2 -> Add1/1, Add/2
  Add1/1 -> Real-Imag to Complex/1
  MatchedIn/1 -> Complex to Real-Imag/1
  Real-Imag to Complex/1 -> Out1/1

== system OFDM_Tx_Rx_InterpDec/OFDMRx/Synchronisation/FineTimingSynch/MatchedFilter/Subsystem35 ==
  MatchedIn : Inport
  Add : Sum  OutDataTypeStr=fixdt(1,18,14)
  Add1 : Sum  Inputs=+-  OutDataTypeStr=fixdt(1,18,14)
  Complex to Real-Imag : ComplexToRealImag
  Real-Imag to Complex : RealImagToComplex
  Unary Minus : UnaryMinus
  Out1 : Outport
  wires:
  Unary Minus/1 -> Real-Imag to Complex/2
  Add/1 -> Unary Minus/1
  Complex to Real-Imag/1 -> Add1/2, Add/1
  Complex to Real-Imag/2 -> Add1/1, Add/2
  Add1/1 -> Real-Imag to Complex/1
  MatchedIn/1 -> Complex to Real-Imag/1
  Real-Imag to Complex/1 -> Out1/1

== system OFDM_Tx_Rx_InterpDec/OFDMRx/Synchronisation/FineTimingSynch/MatchedFilter/Subsystem36 ==
  MatchedIn : Inport
  Add : Sum  OutDataTypeStr=fixdt(1,18,14)
  Add1 : Sum  Inputs=+-  OutDataTypeStr=fixdt(1,18,14)
  Complex to Real-Imag : ComplexToRealImag
  Real-Imag to Complex : RealImagToComplex
  Out1 : Outport
  wires:
  Add/1 -> Real-Imag to Complex/2
  Add1/1 -> Real-Imag to Complex/1
  Complex to Real-Imag/2 -> Add/2, Add1/2
  Complex to Real-Imag/1 -> Add/1, Add1/1
  MatchedIn/1 -> Complex to Real-Imag/1
  Real-Imag to Complex/1 -> Out1/1

== system OFDM_Tx_Rx_InterpDec/OFDMRx/Synchronisation/FineTimingSynch/MatchedFilter/Subsystem37 ==
  MatchedIn : Inport
  Add : Sum  OutDataTypeStr=fixdt(1,18,14)
  Add1 : Sum  Inputs=+-  OutDataTypeStr=fixdt(1,18,14)
  Complex to Real-Imag : ComplexToRealImag
  Real-Imag to Complex : RealImagToComplex
  Unary Minus : UnaryMinus
  Out1 : Outport
  wires:
  Unary Minus/1 -> Real-Imag to Complex/1
  Real-Imag to Complex/1 -> Out1/1
  MatchedIn/1 -> Complex to Real-Imag/1
  Complex to Real-Imag/1 -> Add/1, Add1/1
  Add1/1 -> Real-Imag to Complex/2
  Add/1 -> Unary Minus/1
  Complex to Real-Imag/2 -> Add/2, Add1/2

== system OFDM_Tx_Rx_InterpDec/OFDMRx/Synchronisation/FineTimingSynch/MatchedFilter/Subsystem38 ==
  MatchedIn : Inport
  Add : Sum  OutDataTypeStr=fixdt(1,18,14)
  Add1 : Sum  Inputs=+-  OutDataTypeStr=fixdt(1,18,14)
  Complex to Real-Imag : ComplexToRealImag
  Real-Imag to Complex : RealImagToComplex
  Unary Minus : UnaryMinus
  Out1 : Outport
  wires:
  Unary Minus/1 -> Real-Imag to Complex/1
  Real-Imag to Complex/1 -> Out1/1
  MatchedIn/1 -> Complex to Real-Imag/1
  Complex to Real-Imag/1 -> Add/1, Add1/1
  Add1/1 -> Real-Imag to Complex/2
  Add/1 -> Unary Minus/1
  Complex to Real-Imag/2 -> Add/2, Add1/2

== system OFDM_Tx_Rx_InterpDec/OFDMRx/Synchronisation/FineTimingSynch/MatchedFilter/Subsystem39 ==
  MatchedIn : Inport
  Add : Sum  OutDataTypeStr=fixdt(1,18,14)
  Add1 : Sum  Inputs=+-  OutDataTypeStr=fixdt(1,18,14)
  Complex to Real-Imag : ComplexToRealImag
  Real-Imag to Complex : RealImagToComplex
  Unary Minus : UnaryMinus
  Out1 : Outport
  wires:
  Unary Minus/1 -> Real-Imag to Complex/1
  Real-Imag to Complex/1 -> Out1/1
  MatchedIn/1 -> Complex to Real-Imag/1
  Complex to Real-Imag/1 -> Add/1, Add1/1
  Add1/1 -> Real-Imag to Complex/2
  Add/1 -> Unary Minus/1
  Complex to Real-Imag/2 -> Add/2, Add1/2

== system OFDM_Tx_Rx_InterpDec/OFDMRx/Synchronisation/FineTimingSynch/MatchedFilter/Subsystem4 ==
  MatchedIn : Inport
  Add : Sum  OutDataTypeStr=fixdt(1,18,14)
  Add1 : Sum  Inputs=+-  OutDataTypeStr=fixdt(1,18,14)
  Complex to Real-Imag : ComplexToRealImag
  Real-Imag to Complex : RealImagToComplex
  Out1 : Outport
  wires:
  Real-Imag to Complex/1 -> Out1/1
  MatchedIn/1 -> Complex to Real-Imag/1
  Complex to Real-Imag/1 -> Add/1, Add1/2
  Add1/1 -> Real-Imag to Complex/2
  Add/1 -> Real-Imag to Complex/1
  Complex to Real-Imag/2 -> Add/2, Add1/1

== system OFDM_Tx_Rx_InterpDec/OFDMRx/Synchronisation/FineTimingSynch/MatchedFilter/Subsystem40 ==
  MatchedIn : Inport
  Add : Sum  OutDataTypeStr=fixdt(1,18,14)
  Add1 : Sum  Inputs=+-  OutDataTypeStr=fixdt(1,18,14)
  Complex to Real-Imag : ComplexToRealImag
  Real-Imag to Complex : RealImagToComplex
  Unary Minus : UnaryMinus
  Out1 : Outport
  wires:
  Complex to Real-Imag/2 -> Add1/2, Add/2
  Add/1 -> Unary Minus/1
  Add1/1 -> Real-Imag to Complex/2
  Complex to Real-Imag/1 -> Add1/1, Add/1
  MatchedIn/1 -> Complex to Real-Imag/1
  Real-Imag to Complex/1 -> Out1/1
  Unary Minus/1 -> Real-Imag to Complex/1

== system OFDM_Tx_Rx_InterpDec/OFDMRx/Synchronisation/FineTimingSynch/MatchedFilter/Subsystem41 ==
  MatchedIn : Inport
  Add : Sum  OutDataTypeStr=fixdt(1,18,14)
  Add1 : Sum  Inputs=+-  OutDataTypeStr=fixdt(1,18,14)
  Complex to Real-Imag : ComplexToRealImag
  Real-Imag to Complex : RealImagToComplex
  Unary Minus : UnaryMinus
  Out1 : Outport
  wires:
  Unary Minus/1 -> Real-Imag to Complex/2
  Add/1 -> Unary Minus/1
  Complex to Real-Imag/1 -> Add1/2, Add/1
  Complex to Real-Imag/2 -> Add1/1, Add/2
  Add1/1 -> Real-Imag to Complex/1
  MatchedIn/1 -> Complex to Real-Imag/1
  Real-Imag to Complex/1 -> Out1/1

== system OFDM_Tx_Rx_InterpDec/OFDMRx/Synchronisation/FineTimingSynch/MatchedFilter/Subsystem42 ==
  MatchedIn : Inport
  Add : Sum  OutDataTypeStr=fixdt(1,18,14)
  Add1 : Sum  Inputs=+-  OutDataTypeStr=fixdt(1,18,14)
  Complex to Real-Imag : ComplexToRealImag
  Real-Imag to Complex : RealImagToComplex
  Out1 : Outport
  wires:
  Real-Imag to Complex/1 -> Out1/1
  MatchedIn/1 -> Complex to Real-Imag/1
  Complex to Real-Imag/1 -> Add/1, Add1/2
  Add1/1 -> Real-Imag to Complex/2
  Add/1 -> Real-Imag to Complex/1
  Complex to Real-Imag/2 -> Add/2, Add1/1

== system OFDM_Tx_Rx_InterpDec/OFDMRx/Synchronisation/FineTimingSynch/MatchedFilter/Subsystem43 ==
  MatchedIn : Inport
  Add : Sum  OutDataTypeStr=fixdt(1,18,14)
  Add1 : Sum  Inputs=+-  OutDataTypeStr=fixdt(1,18,14)
  Complex to Real-Imag : ComplexToRealImag
  Real-Imag to Complex : RealImagToComplex
  Out1 : Outport
  wires:
  Real-Imag to Complex/1 -> Out1/1
  MatchedIn/1 -> Complex to Real-Imag/1
  Complex to Real-Imag/1 -> Add/1, Add1/2
  Add1/1 -> Real-Imag to Complex/2
  Add/1 -> Real-Imag to Complex/1
  Complex to Real-Imag/2 -> Add/2, Add1/1

== system OFDM_Tx_Rx_InterpDec/OFDMRx/Synchronisation/FineTimingSynch/MatchedFilter/Subsystem44 ==
  MatchedIn : Inport
  Add : Sum  OutDataTypeStr=fixdt(1,18,14)
  Add1 : Sum  Inputs=+-  OutDataTypeStr=fixdt(1,18,14)
  Complex to Real-Imag : ComplexToRealImag
  Real-Imag to Complex : RealImagToComplex
  Unary Minus : UnaryMinus
  Out1 : Outport
  wires:
  Real-Imag to Complex/1 -> Out1/1
  MatchedIn/1 -> Complex to Real-Imag/1
  Add1/1 -> Real-Imag to Complex/1
  Complex to Real-Imag/2 -> Add/2, Add1/1
  Complex to Real-Imag/1 -> Add/1, Add1/2
  Add/1 -> Unary Minus/1
  Unary Minus/1 -> Real-Imag to Complex/2

== system OFDM_Tx_Rx_InterpDec/OFDMRx/Synchronisation/FineTimingSynch/MatchedFilter/Subsystem45 ==
  MatchedIn : Inport
  Add : Sum  OutDataTypeStr=fixdt(1,18,14)
  Add1 : Sum  Inputs=+-  OutDataTypeStr=fixdt(1,18,14)
  Complex to Real-Imag : ComplexToRealImag
  Real-Imag to Complex : RealImagToComplex
  Unary Minus : UnaryMinus
  Out1 : Outport
  wires:
  Unary Minus/1 -> Real-Imag to Complex/2
  Add/1 -> Unary Minus/1
  Complex to Real-Imag/1 -> Add1/2, Add/1
  Complex to Real-Imag/2 -> Add1/1, Add/2
  Add1/1 -> Real-Imag to Complex/1
  MatchedIn/1 -> Complex to Real-Imag/1
  Real-Imag to Complex/1 -> Out1/1

== system OFDM_Tx_Rx_InterpDec/OFDMRx/Synchronisation/FineTimingSynch/MatchedFilter/Subsystem46 ==
  MatchedIn : Inport
  Add : Sum  OutDataTypeStr=fixdt(1,18,14)
  Add1 : Sum  Inputs=+-  OutDataTypeStr=fixdt(1,18,14)
  Complex to Real-Imag : ComplexToRealImag
  Real-Imag to Complex : RealImagToComplex
  Out1 : Outport
  wires:
  Real-Imag to Complex/1 -> Out1/1
  MatchedIn/1 -> Complex to Real-Imag/1
  Complex to Real-Imag/1 -> Add/1, Add1/2
  Add1/1 -> Real-Imag to Complex/2
  Add/1 -> Real-Imag to Complex/1
  Complex to Real-Imag/2 -> Add/2, Add1/1

== system OFDM_Tx_Rx_InterpDec/OFDMRx/Synchronisation/FineTimingSynch/MatchedFilter/Subsystem47 ==
  MatchedIn : Inport
  Add : Sum  OutDataTypeStr=fixdt(1,18,14)
  Add1 : Sum  Inputs=+-  OutDataTypeStr=fixdt(1,18,14)
  Complex to Real-Imag : ComplexToRealImag
  Real-Imag to Complex : RealImagToComplex
  Out1 : Outport
  wires:
  Add/1 -> Real-Imag to Complex/2
  Add1/1 -> Real-Imag to Complex/1
  Complex to Real-Imag/2 -> Add/2, Add1/2
  Complex to Real-Imag/1 -> Add/1, Add1/1
  MatchedIn/1 -> Complex to Real-Imag/1
  Real-Imag to Complex/1 -> Out1/1

== system OFDM_Tx_Rx_InterpDec/OFDMRx/Synchronisation/FineTimingSynch/MatchedFilter/Subsystem48 ==
  MatchedIn : Inport
  Add : Sum  OutDataTypeStr=fixdt(1,18,14)
  Add1 : Sum  Inputs=+-  OutDataTypeStr=fixdt(1,18,14)
  Complex to Real-Imag : ComplexToRealImag
  Real-Imag to Complex : RealImagToComplex
  Out1 : Outport
  wires:
  Real-Imag to Complex/1 -> Out1/1
  MatchedIn/1 -> Complex to Real-Imag/1
  Complex to Real-Imag/1 -> Add1/1, Add/1
  Complex to Real-Imag/2 -> Add1/2, Add/2
  Add1/1 -> Real-Imag to Complex/1
  Add/1 -> Real-Imag to Complex/2

== system OFDM_Tx_Rx_InterpDec/OFDMRx/Synchronisation/FineTimingSynch/MatchedFilter/Subsystem5 ==
  MatchedIn : Inport
  Add : Sum  OutDataTypeStr=fixdt(1,18,14)
  Add1 : Sum  Inputs=+-  OutDataTypeStr=fixdt(1,18,14)
  Complex to Real-Imag : ComplexToRealImag
  Real-Imag to Complex : RealImagToComplex
  Unary Minus : UnaryMinus
  Out1 : Outport
  wires:
  Unary Minus/1 -> Real-Imag to Complex/2
  Add/1 -> Unary Minus/1
  Complex to Real-Imag/1 -> Add1/2, Add/1
  Complex to Real-Imag/2 -> Add1/1, Add/2
  Add1/1 -> Real-Imag to Complex/1
  MatchedIn/1 -> Complex to Real-Imag/1
  Real-Imag to Complex/1 -> Out1/1

== system OFDM_Tx_Rx_InterpDec/OFDMRx/Synchronisation/FineTimingSynch/MatchedFilter/Subsystem50 ==
  MatchedIn : Inport
  Add : Sum  OutDataTypeStr=fixdt(1,18,14)
  Add1 : Sum  Inputs=+-  OutDataTypeStr=fixdt(1,18,14)
  Complex to Real-Imag : ComplexToRealImag
  Real-Imag to Complex : RealImagToComplex
  Out1 : Outport
  wires:
  Add/1 -> Real-Imag to Complex/2
  Add1/1 -> Real-Imag to Complex/1
  Complex to Real-Imag/2 -> Add/2, Add1/2
  Complex to Real-Imag/1 -> Add/1, Add1/1
  MatchedIn/1 -> Complex to Real-Imag/1
  Real-Imag to Complex/1 -> Out1/1

== system OFDM_Tx_Rx_InterpDec/OFDMRx/Synchronisation/FineTimingSynch/MatchedFilter/Subsystem51 ==
  MatchedIn : Inport
  Add : Sum  OutDataTypeStr=fixdt(1,18,14)
  Add1 : Sum  Inputs=+-  OutDataTypeStr=fixdt(1,18,14)
  Complex to Real-Imag : ComplexToRealImag
  Real-Imag to Complex : RealImagToComplex
  Out1 : Outport
  wires:
  Real-Imag to Complex/1 -> Out1/1
  MatchedIn/1 -> Complex to Real-Imag/1
  Complex to Real-Imag/1 -> Add1/1, Add/1
  Complex to Real-Imag/2 -> Add1/2, Add/2
  Add1/1 -> Real-Imag to Complex/1
  Add/1 -> Real-Imag to Complex/2

== system OFDM_Tx_Rx_InterpDec/OFDMRx/Synchronisation/FineTimingSynch/MatchedFilter/Subsystem52 ==
  MatchedIn : Inport
  Add : Sum  OutDataTypeStr=fixdt(1,18,14)
  Add1 : Sum  Inputs=+-  OutDataTypeStr=fixdt(1,18,14)
  Complex to Real-Imag : ComplexToRealImag
  Real-Imag to Complex : RealImagToComplex
  Unary Minus : UnaryMinus
  Out1 : Outport
  wires:
  Unary Minus/1 -> Real-Imag to Complex/1
  Real-Imag to Complex/1 -> Out1/1
  MatchedIn/1 -> Complex to Real-Imag/1
  Complex to Real-Imag/1 -> Add/1, Add1/1
  Add1/1 -> Real-Imag to Complex/2
  Add/1 -> Unary Minus/1
  Complex to Real-Imag/2 -> Add/2, Add1/2

== system OFDM_Tx_Rx_InterpDec/OFDMRx/Synchronisation/FineTimingSynch/MatchedFilter/Subsystem53 ==
  MatchedIn : Inport
  Add : Sum  OutDataTypeStr=fixdt(1,18,14)
  Add1 : Sum  Inputs=+-  OutDataTypeStr=fixdt(1,18,14)
  Complex to Real-Imag : ComplexToRealImag
  Real-Imag to Complex : RealImagToComplex
  Out1 : Outport
  wires:
  Add/1 -> Real-Imag to Complex/2
  Add1/1 -> Real-Imag to Complex/1
  Complex to Real-Imag/2 -> Add/2, Add1/2
  Complex to Real-Imag/1 -> Add/1, Add1/1
  MatchedIn/1 -> Complex to Real-Imag/1
  Real-Imag to Complex/1 -> Out1/1

== system OFDM_Tx_Rx_InterpDec/OFDMRx/Synchronisation/FineTimingSynch/MatchedFilter/Subsystem54 ==
  MatchedIn : Inport
  Add : Sum  OutDataTypeStr=fixdt(1,18,14)
  Add1 : Sum  Inputs=+-  OutDataTypeStr=fixdt(1,18,14)
  Complex to Real-Imag : ComplexToRealImag
  Real-Imag to Complex : RealImagToComplex
  Out1 : Outport
  wires:
  Real-Imag to Complex/1 -> Out1/1
  MatchedIn/1 -> Complex to Real-Imag/1
  Complex to Real-Imag/1 -> Add/1, Add1/2
  Add1/1 -> Real-Imag to Complex/2
  Add/1 -> Real-Imag to Complex/1
  Complex to Real-Imag/2 -> Add/2, Add1/1

== system OFDM_Tx_Rx_InterpDec/OFDMRx/Synchronisation/FineTimingSynch/MatchedFilter/Subsystem55 ==
  MatchedIn : Inport
  Add : Sum  OutDataTypeStr=fixdt(1,18,14)
  Add1 : Sum  Inputs=+-  OutDataTypeStr=fixdt(1,18,14)
  Complex to Real-Imag : ComplexToRealImag
  Real-Imag to Complex : RealImagToComplex
  Out1 : Outport
  wires:
  Add/1 -> Real-Imag to Complex/2
  Add1/1 -> Real-Imag to Complex/1
  Complex to Real-Imag/2 -> Add/2, Add1/2
  Complex to Real-Imag/1 -> Add/1, Add1/1
  MatchedIn/1 -> Complex to Real-Imag/1
  Real-Imag to Complex/1 -> Out1/1

== system OFDM_Tx_Rx_InterpDec/OFDMRx/Synchronisation/FineTimingSynch/MatchedFilter/Subsystem56 ==
  MatchedIn : Inport
  Add : Sum  OutDataTypeStr=fixdt(1,18,14)
  Add1 : Sum  Inputs=+-  OutDataTypeStr=fixdt(1,18,14)
  Complex to Real-Imag : ComplexToRealImag
  Real-Imag to Complex : RealImagToComplex
  Unary Minus : UnaryMinus
  Out1 : Outport
  wires:
  Unary Minus/1 -> Real-Imag to Complex/1
  Real-Imag to Complex/1 -> Out1/1
  MatchedIn/1 -> Complex to Real-Imag/1
  Complex to Real-Imag/1 -> Add/1, Add1/1
  Add1/1 -> Real-Imag to Complex/2
  Add/1 -> Unary Minus/1
  Complex to Real-Imag/2 -> Add/2, Add1/2

== system OFDM_Tx_Rx_InterpDec/OFDMRx/Synchronisation/FineTimingSynch/MatchedFilter/Subsystem57 ==
  MatchedIn : Inport
  Add : Sum  OutDataTypeStr=fixdt(1,18,14)
  Add1 : Sum  Inputs=+-  OutDataTypeStr=fixdt(1,18,14)
  Complex to Real-Imag : ComplexToRealImag
  Real-Imag to Complex : RealImagToComplex
  Unary Minus : UnaryMinus
  Out1 : Outport
  wires:
  Unary Minus/1 -> Real-Imag to Complex/1
  Real-Imag to Complex/1 -> Out1/1
  MatchedIn/1 -> Complex to Real-Imag/1
  Complex to Real-Imag/1 -> Add/1, Add1/1
  Add1/1 -> Real-Imag to Complex/2
  Add/1 -> Unary Minus/1
  Complex to Real-Imag/2 -> Add/2, Add1/2

== system OFDM_Tx_Rx_InterpDec/OFDMRx/Synchronisation/FineTimingSynch/MatchedFilter/Subsystem58 ==
  MatchedIn : Inport
  Add : Sum  OutDataTypeStr=fixdt(1,18,14)
  Add1 : Sum  Inputs=+-  OutDataTypeStr=fixdt(1,18,14)
  Complex to Real-Imag : ComplexToRealImag
  Real-Imag to Complex : RealImagToComplex
  Out1 : Outport
  wires:
  Add/1 -> Real-Imag to Complex/2
  Add1/1 -> Real-Imag to Complex/1
  Complex to Real-Imag/2 -> Add/2, Add1/2
  Complex to Real-Imag/1 -> Add/1, Add1/1
  MatchedIn/1 -> Complex to Real-Imag/1
  Real-Imag to Complex/1 -> Out1/1
